simulink model "lab9"  (R2014b)
settings: Solver=ode45  StartTime=0.0  StopTime=15  MaxStep=0.001  MinStep=0.0001  RelTol=1e-3
values from neighbouring files (symbols this model uses):
  k = 2    [lab9.mat]
  T = 0.5    [lab9.mat]
settings Model: Creator=Игорь  LastModifiedBy=Игорь

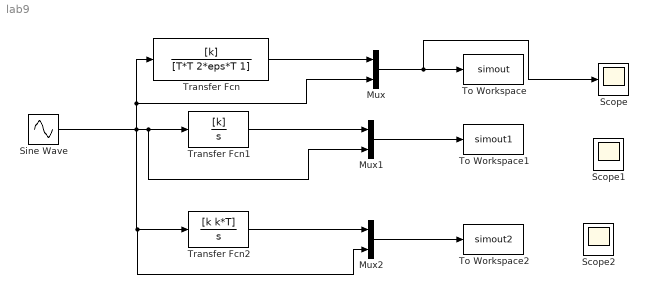
== system lab9 ==
  Mux : Mux  Inputs=2
  Mux1 : Mux  Inputs=2
  Mux2 : Mux  Inputs=2
  Scope : Scope
  Scope1 : Scope
  Scope2 : Scope
      settings: SaveName=ScopeData2
  Sine Wave : Sin  Frequency=5  SampleTime=0
  To Workspace : ToWorkspace  VariableName=simout  SaveFormat=Timeseries  SampleTime=-1
  To Workspace1 : ToWorkspace  VariableName=simout1  SaveFormat=Timeseries  SampleTime=-1
  To Workspace2 : ToWorkspace  VariableName=simout2  SaveFormat=Timeseries  SampleTime=-1
  Transfer Fcn : TransferFcn  Numerator=[k]  Denominator=[T*T 2*eps*T 1]
  Transfer Fcn1 : TransferFcn  Numerator=[k]  Denominator=[1 0]
  Transfer Fcn2 : TransferFcn  Numerator=[k k*T]  Denominator=[1 0]
  wires:
  Transfer Fcn/1 -> Mux/1
  Sine Wave/1 -> Transfer Fcn/1, Mux/2, Mux2/2, Transfer Fcn2/1, Mux1/2, Transfer Fcn1/1
  Transfer Fcn1/1 -> Mux1/1
  Mux/1 -> Scope/1, To Workspace/1
  Mux1/1 -> To Workspace1/1
  Mux2/1 -> To Workspace2/1
  Transfer Fcn2/1 -> Mux2/1
